simulink model "logical_operations"  (R2024b)
settings: Solver=ode3  StartTime=0.0  StopTime=10.0  FixedStep=0.01  RelTol=1e-3
libraries: simulink x1
settings Model: Creator=balaj  LastModifiedBy=balaj

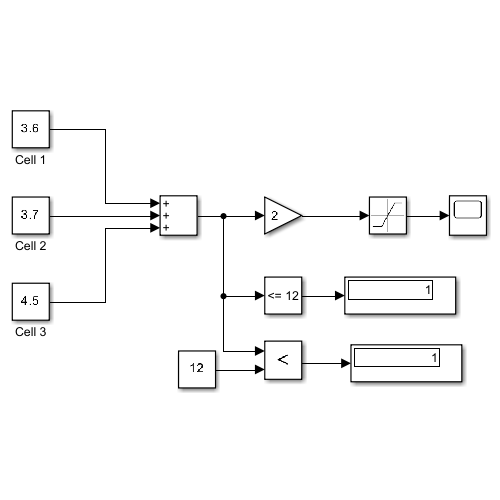
[thumbnail: Simulink's stored preview of the top-level diagram]
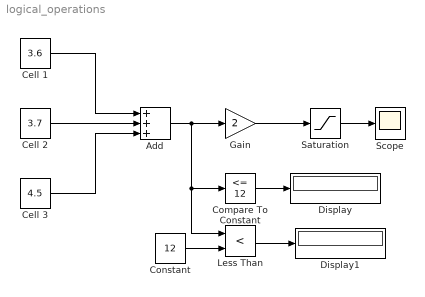
== system logical_operations ==
  Add : Sum  Inputs=+++
  Cell 1 : Constant  Value=3.6  SampleTime=1
  Cell 2 : Constant  Value=3.7  SampleTime=1
  Cell 3 : Constant  Value=4.5  SampleTime=1
  Compare To Constant : simulink/Logic and Bit Operations/Compare To Constant  relop=<=  const=12  OutDataTypeStr=boolean
  Constant : Constant  Value=12
  Display : Display
  Display1 : Display
  Gain : Gain  Gain=2
  Less Than : RelationalOperator  Operator=<  OutDataTypeStr=boolean  RndMeth=Simplest  InputSameDT=off
  Saturation : Saturate  UpperLimit=12  LowerLimit=0
  Scope : Scope
  wires:
  Cell 1/1 -> Add/1
  Cell 2/1 -> Add/2
  Cell 3/1 -> Add/3
  Add/1 -> Less Than/1, Compare To Constant/1, Gain/1
  Gain/1 -> Saturation/1
  Saturation/1 -> Scope/1
  Compare To Constant/1 -> Display/1
  Constant/1 -> Less Than/2
  Less Than/1 -> Display1/1
